simulink model "hu_flatness"  (R2017b)
settings: Solver=VariableStepAuto  StartTime=0.0  StopTime=102  RelTol=1e-9
libraries: simulink x1
(part 1 of 3)
settings Model: Creator=chenjiasheng  LastModifiedBy=chenjiasheng

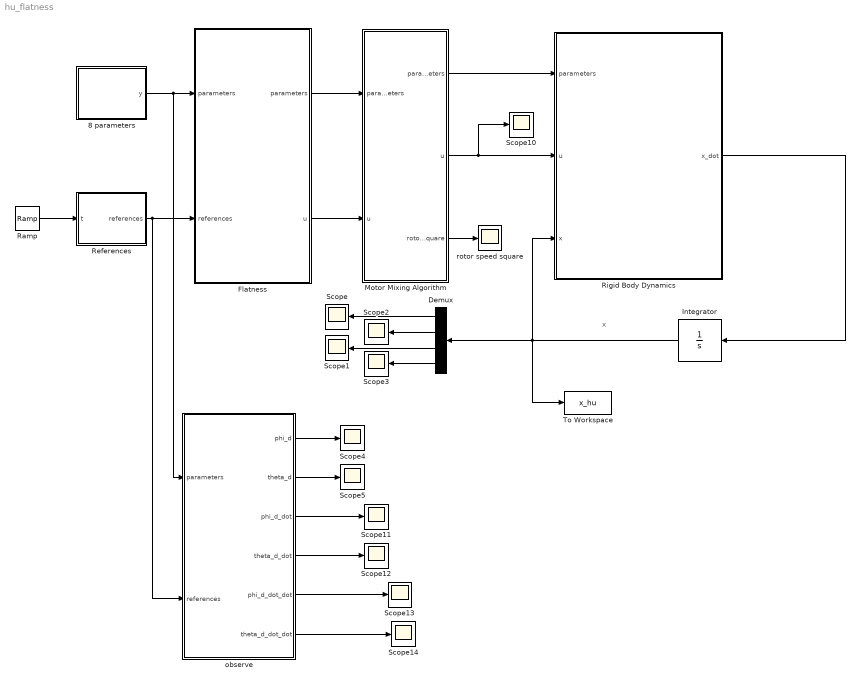
== system hu_flatness ==
  note: x
  8 parameters : MATLAB Function  TreatAsAtomicUnit=on
  Demux : Demux
  Flatness : MATLAB Function  TreatAsAtomicUnit=on
  Integrator : Integrator  InitialCondition=x_xi4(end,:)  ContinuousStateAttributes='x'
  Motor Mixing Algorithm : MATLAB Function  TreatAsAtomicUnit=on
  Ramp : simulink/Sources/Ramp  slope=1  start=0  X0=0
  References : MATLAB Function  TreatAsAtomicUnit=on
  Rigid Body Dynamics : MATLAB Function  TreatAsAtomicUnit=on
  Scope{,1..5,10..14} (11 alike) : Scope
  To Workspace : ToWorkspace  VariableName=x_hu  SampleTime=0.01
  observe : MATLAB Function  TreatAsAtomicUnit=on
  rotor speed square : Scope
  wires:
  Rigid Body Dynamics/1(x_dot) -> Integrator/1
  Motor Mixing Algorithm/3(rotor_speed_square) -> rotor speed square/1
  Motor Mixing Algorithm/1(parameters) -> Rigid Body Dynamics/1(parameters)
  Integrator/1 -> To Workspace/1, Demux/1, Rigid Body Dynamics/3(x)
  Motor Mixing Algorithm/2(u) -> Scope10/1, Rigid Body Dynamics/2(u)
  Ramp/1 -> References/1(t)
  Flatness/1(parameters) -> Motor Mixing Algorithm/1("parameters ")
  Flatness/2(u) -> Motor Mixing Algorithm/2("u ")
  References/1(references) -> Flatness/2(references), observe/2(references)
  8 parameters/1(y) -> Flatness/1("parameters "), observe/1(parameters)
  Demux/1 -> Scope/1
  Demux/3 -> Scope1/1
  Demux/2 -> Scope2/1
  Demux/4 -> Scope3/1
  observe/3(phi_d_dot) -> Scope11/1
  observe/4(theta_d_dot) -> Scope12/1
  observe/5(phi_d_dot_dot) -> Scope13/1
  observe/6(theta_d_dot_dot) -> Scope14/1
  observe/1(phi_d) -> Scope4/1
  observe/2(theta_d) -> Scope5/1

== matlab function hu_flatness/Flatness ==
  data: parameters input; parameters output; references input; u output
function [parameters, u] = fcn(parameters,references)
% allocate input
m=parameters(1);
g=parameters(2);
M=diag(parameters(3:5));
r_d=references(1:3) ;          % reference's positions
r_d_dot=references(4:6);       % reference's velocities
a_d=references(7:9) ;          % reference's accelerations
a_d_dot=references(10:12);     % jerk
a_d_dot_dot=references(13:15); % snap
psi_d=references(16);          % reference's yaw angle 
psi_d_dot=references(17);
psi_d_dot_dot=references(18);

%% define some variables to make your life easier (f is not artifically defined)
f=m*sqrt(a_d(1)^2+a_d(2)^2+(g+a_d(3))^2);    % f is  the 1st element of input u
C=a_d(1)*cos(psi_d)+a_d(2)*sin(psi_d);      %
D=g+a_d(3);                                 %
A=a_d(1)*sin(psi_d)-a_d(2)*cos(psi_d);      %
B=sqrt(C^2+D^2);                            %
A_dot=sin(psi_d)*a_d_dot(1)-cos(psi_d)*a_d_dot(2)+C*psi_d_dot;                                   %
C_dot=cos(psi_d)*a_d_dot(1)+sin(psi_d)*a_d_dot(2)-A*psi_d_dot;                                   %
D_dot=a_d_dot(3);                                                                                %
B_dot=(C*C_dot+D*D_dot)/B;  
fbmsd=2*a_d(1)*a_d_dot(1)+2*a_d(2)*a_d_dot(2)+2*(g+a_d(3))*a_d_dot(3);   % f by m square dot
%% phi_d, theta_d
phi_d=asin(A*m/f) ;
if C>0
theta_d=acos(D/B) ;
else
theta_d=-acos(D/B) ;
end
%% phi_d_dot, theta_d_dot
phi_d_dot=(sin(psi_d)*(f/m)^2-A*a_d(1))/((f/m)^2*B)*a_d_dot(1) + (-cos(psi_d)*(f/m)^2-A*a_d(2))/((f/m)^2*B)*a_d_dot(2) + (-A*D)/((f/m)^2*B)*a_d_dot(3) + C/B*psi_d_dot;
theta_d_dot=(cos(psi_d)*D*a_d_dot(1)+sin(psi_d)*D*a_d_dot(2)-C*a_d_dot(3)-A*D*psi_d_dot)/B^2   ;

%% phi_d_dot_dot, theta_d_dot_dot
monster11=(cos(psi_d)*psi_d_dot*(f/m)^2+sin(psi_d)*fbmsd-(A_dot*a_d(1)+A*a_d_dot(1)))*a_d_dot(1)+(sin(psi_d)*(f/m)^2-A*a_d(1))*a_d_dot_dot(1);
monster12=(-sin(psi_d)*psi_d_dot*(f/m)^2+cos(psi_d)*fbmsd+A_dot*a_d(2)+A*a_d_dot(2))*a_d_dot(2)+(cos(psi_d)*(f/m)^2+A*a_d(2))*a_d_dot_dot(2);
monster13=(A_dot*D+A*D_dot)*a_d_dot(3)+A*D*a_d_dot_dot(3);
monster1=monster11-monster12-monster13;
phi_d_dot_dot=(monster1-(B*phi_d_dot-C*psi_d_dot)*fbmsd)/((f/m)^2*B) + (C_dot*psi_d_dot+C*psi_d_dot_dot-B_dot*phi_d_dot)/B;
monster21=(-sin(psi_d)*psi_d_dot*D+cos(psi_d)*D_dot)*a_d_dot(1)+cos(psi_d)*D*a_d_dot_dot(1);
monster22=(cos(psi_d)*psi_d_dot*D+sin(psi_d)*D_dot)*a_d_dot(2)+sin(psi_d)*D*a_d_dot_dot(2);
monster23= C_dot*a_d_dot(3)+C*a_d_dot_dot(3);
monster24=(A_dot*D+A*D_dot)*psi_d_dot+A*D*psi_d_dot_dot;
monster2= monster21+monster22-monster23-monster24;
theta_d_dot_dot=monster2/B^2-2*theta_d_dot*B_dot/B;

%% omegab, omegab_dot
Lnb=[1 0           -sin(theta_d);
     0 cos(phi_d)  sin(phi_d)*cos(theta_d);
     0 -sin(phi_d) cos(phi_d)*cos(theta_d)];
omegab=Lnb*[phi_d_dot;theta_d_dot;psi_d_dot];
omegab_dot=Lnb*[phi_d_dot_dot;theta_d_dot_dot;psi_d_dot_dot]+[-cos(theta_d)            0                        0;
                                                              -sin(phi_d)*sin(theta_d) cos(phi_d)*cos(theta_d)  -sin(phi_d);
                                                              -cos(phi_d)*sin(theta_d) -sin(phi_d)*cos(theta_d) -cos(phi_d)]*[theta_d_dot*psi_d_dot;phi_d_dot*psi_d_dot;phi_d_dot*theta_d_dot];

%% taub,u
taub=M*omegab_dot+cross(omegab,M*omegab);
u=[f;taub];
end

== matlab function hu_flatness/8 parameters ==
  data: y output size=8
function y=fcn
%% specify parameters
m=0.468;
g=9.81;
Ix=4.856*10^(-3);
Iy=4.856*10^(-3);
Iz=8.801*10^(-3);
l=0.225;
k=2.980*10^-6;
c=1.140*10^-7;
%% output
y=[m;g;Ix;Iy;Iz;l;k;c] ;% output # 1-8
    
end

== matlab function hu_flatness/observe ==
  data: parameters input; phi_d output; references input; theta_d output; phi_d_dot output; theta_d_dot output; phi_d_dot_dot output; theta_d_dot_dot output
function [phi_d,theta_d,phi_d_dot,theta_d_dot,phi_d_dot_dot,theta_d_dot_dot] = fcn(parameters,references)
% allocate input
m=parameters(1);
g=parameters(2);
M=diag(parameters(3:5));
r_d=references(1:3) ;          % reference's positions
r_d_dot=references(4:6);       % reference's velocities
a_d=references(7:9) ;          % reference's accelerations
a_d_dot=references(10:12);     % jerk
a_d_dot_dot=references(13:15); % snap
psi_d=references(16);          % reference's yaw angle 
psi_d_dot=references(17);
psi_d_dot_dot=references(18);

%% define some variables to make your life easier (f is not artifically defined)
f=m*sqrt(a_d(1)^2+a_d(2)^2+(g+a_d(3))^2);    % f is  the 1st element of input u
C=a_d(1)*cos(psi_d)+a_d(2)*sin(psi_d);      %
D=g+a_d(3);                                 %
A=a_d(1)*sin(psi_d)-a_d(2)*cos(psi_d);      %
B=sqrt(C^2+D^2);                            %
A_dot=sin(psi_d)*a_d_dot(1)-cos(psi_d)*a_d_dot(2)+C*psi_d_dot;                                   %   
C_dot=cos(psi_d)*a_d_dot(1)+sin(psi_d)*a_d_dot(2)-A*psi_d_dot;                                   %
D_dot=a_d_dot(3);                                                                                %
B_dot=(C*C_dot+D*D_dot)/B;
fbmsd=2*a_d(1)*a_d_dot(1)+2*a_d(2)*a_d_dot(2)+2*(g+a_d(3))*a_d_dot(3);   % f by m square dot
%% phi_d, theta_d
phi_d=asin(A*m/f) ;
if C>0
theta_d=acos(D/B) ;
else
theta_d=-acos(D/B) ;
end
%% phi_d_dot, theta_d_dot
phi_d_dot=(sin(psi_d)*(f/m)^2-A*a_d(1))/((f/m)^2*B)*a_d_dot(1) + (-cos(psi_d)*(f/m)^2-A*a_d(2))/((f/m)^2*B)*a_d_dot(2) + (-A*D)/((f/m)^2*B)*a_d_dot(3) + C/B*psi_d_dot;
theta_d_dot=(cos(psi_d)*D*a_d_dot(1)+sin(psi_d)*D*a_d_dot(2)-C*a_d_dot(3)-A*D*psi_d_dot)/B^2   ;

%% phi_d_dot_dot, theta_d_dot_dot
monster11=(cos(psi_d)*psi_d_dot*(f/m)^2+sin(psi_d)*fbmsd-(A_dot*a_d(1)+A*a_d_dot(1)))*a_d_dot(1)+(sin(psi_d)*(f/m)^2-A*a_d(1))*a_d_dot_dot(1);
monster12=(-sin(psi_d)*psi_d_dot*(f/m)^2+cos(psi_d)*fbmsd+A_dot*a_d(2)+A*a_d_dot(2))*a_d_dot(2)+(cos(psi_d)*(f/m)^2+A*a_d(2))*a_d_dot_dot(2);
monster13=(A_dot*D+A*D_dot)*a_d_dot(3)+A*D*a_d_dot_dot(3);
monster1=monster11-monster12-monster13;
phi_d_dot_dot=(monster1-(B*phi_d_dot-C*psi_d_dot)*fbmsd)/((f/m)^2*B) + (C_dot*psi_d_dot+C*psi_d_dot_dot-B_dot*phi_d_dot)/B;
monster21=(-sin(psi_d)*psi_d_dot*D+cos(psi_d)*D_dot)*a_d_dot(1)+cos(psi_d)*D*a_d_dot_dot(1);
monster22=(cos(psi_d)*psi_d_dot*D+sin(psi_d)*D_dot)*a_d_dot(2)+sin(psi_d)*D*a_d_dot_dot(2);
monster23= C_dot*a_d_dot(3)+C*a_d_dot_dot(3);
monster24=(A_dot*D+A*D_dot)*psi_d_dot+A*D*psi_d_dot_dot;
monster2= monster21+monster22-monster23-monster24;
theta_d_dot_dot=monster2/B^2-2*theta_d_dot*B_dot/B;

%% omegab, omegab_dot
Lnb=[1 0           -sin(theta_d);
     0 cos(phi_d)  sin(phi_d)*cos(theta_d);
     0 -sin(phi_d) cos(phi_d)*cos(theta_d)];
omegab=Lnb*[phi_d_dot;theta_d_dot;psi_d_dot];
omegab_dot=Lnb*[phi_d_dot_dot;theta_d_dot_dot;psi_d_dot_dot]+[-cos(theta_d)            0                        0;
                                                              -sin(phi_d)*sin(theta_d) cos(phi_d)*cos(theta_d)  -sin(phi_d);
                                                              -cos(phi_d)*sin(theta_d) -sin(phi_d)*cos(theta_d) -cos(phi_d)]*[theta_d_dot*psi_d_dot;phi_d_dot*psi_d_dot;phi_d_dot*theta_d_dot];

%% taub,u
taub=M*omegab_dot+cross(omegab,M*omegab);
u=[f;taub];
end
